simulink model "PrinterMotorP"  (R2015b)
settings: Solver=VariableStepAuto  StartTime=0.0  StopTime=10.0  RelTol=1e-3
libraries: fuzblock x1
settings Model: Creator=Christian Dos Santos  LastModifiedBy=Christian Dos Santos

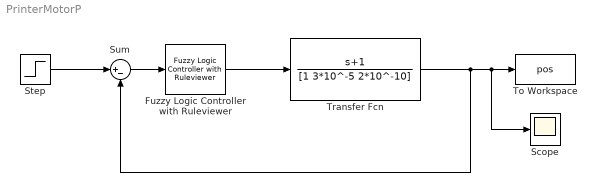
== system PrinterMotorP ==
  Fuzzy Logic Controller with Ruleviewer : fuzblock/Fuzzy Logic  Controller  with Ruleviewer  fismatrix=PrinterMotor  Ts=2
  Scope : Scope
  Step : Step  After=10  SampleTime=0
  Sum : Sum  Inputs=|+-
  To Workspace : ToWorkspace  VariableName=pos  SampleTime=-1
  Transfer Fcn : TransferFcn  Numerator=[1 1]  Denominator=[1 3*10^-5 2*10^-10]
  wires:
  Fuzzy Logic Controller with Ruleviewer/1 -> Transfer Fcn/1
  Sum/1 -> Fuzzy Logic Controller with Ruleviewer/1
  Step/1 -> Sum/1
  Transfer Fcn/1 -> Scope/1, To Workspace/1, Sum/2
